simulink model "AngleSpeedToPWM"  (R2017b)
settings: Solver=FixedStepDiscrete  StartTime=0.0  StopTime=5000  FixedStep=1  RelTol=1e-3
libraries: simulink x1, hdlsllib x1
settings Model: Creator=chandler.ga  LastModifiedBy=Gavin
settings CodeAppCC: StateflowObjectComments=on

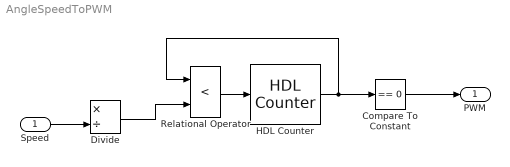
== system AngleSpeedToPWM ==
  Speed : Inport
  Compare To Constant : simulink/Logic and Bit Operations/Compare To Constant  relop===  const=0  OutDataTypeStr=boolean
  Divide : Product  Inputs=*/  SaturateOnIntegerOverflow=on  RndMeth=Zero
  HDL Counter : hdlsllib/Sources/HDL Counter  CountType=Count limited  CountInit=0  CountStep=1  CountMax=1000  CountFromType=Initial value  CountFrom=0  CountResetPort=on  CountLoadPort=off  CountEnbPort=off  CountDirPort=off  CountDataType=Unsigned  CountWordLen=10  CountFracLen=0  CountSampTime=1
      settings: SourceProductBaseCode=HD
  Relational Operator : RelationalOperator  Operator=<  OutDataTypeStr=boolean  RndMeth=Nearest
  PWM : Outport
  wires:
  HDL Counter/1 -> Relational Operator/1, Compare To Constant/1
  Compare To Constant/1 -> PWM/1
  Relational Operator/1 -> HDL Counter/1
  Divide/1 -> Relational Operator/2
  Speed/1 -> Divide/2
